simulink model "cont2_nrz_v8"  (R2016b)
settings: Solver=ode23t  StartTime=0.0  StopTime=L  FixedStep=1  RelTol=1e-6  AbsTol=1e-6
values from neighbouring files (symbols this model uses):
  a = amp(compt)    [QPSK.m]
  fin = fin_bin/Nfft    (= 0.00079345703125)    [DS_TB.m]    (also in Trace_RC.m)
settings Model: ExtModeTrigMode=oneshot  ExtModeArmWhenConnect=off  ExtModeAutoUpdateStatusClock=off  Creator=sigma  LastModifiedBy=charles
settings DataIOCC: SaveFormat=Array  SignalLoggingSaveFormat=ModelDataLogs  SaveOutput=off  SaveTime=off  SignalLoggingName=sigsOut
settings OptimizationCC: BooleanDataType=off  ExpressionDepthLimit=2147483647  InitFltsAndDblsToZero=on  LifeSpan=inf
settings DebuggingCC: SaveWithParameterizedLinksMsg=none  UnderspecifiedInitializationDetection=Classic  MergeDetectMultiDrivingBlocksExec=none  SignalResolutionControl=TryResolveAllWithWarning  MultiTaskDSMMsg=warning  MultiTaskCondExecSysMsg=none  FcnCallInpInsideContextMsg=warning  StateNameClashWarn=warning  SFUnexpectedBacktrackingDiag=warning  SFNoUnconditionalDefaultTransitionDiag=warning  SFExecutionAtInitializationDiag=none
settings HardwareCC: ProdBitPerPointer=32  ProdBitPerSizeT=32  ProdBitPerPtrDiffT=32  ProdLargestAtomicFloat=None  ProdIntDivRoundTo=Undefined  ProdEndianess=Unspecified  ProdWordSize=32  ProdHWDeviceType=32-bit Generic  TargetUnknown=on
settings ModelReferenceCC: PropagateSignalLabelsOutOfModel=off
settings RTWCC: TemplateMakefile=grt_unix.tmf
settings GRTTargetCC: TargetLangStandard=C89/C90 (ANSI)  ModelReferenceCompliant=off  ParMdlRefBuildCompliant=off  CompOptLevelCompliant=off  ConcurrentExecutionCompliant=off  CombineOutputUpdateFcns=off  MatFileLogging=off  MATLABClassNameForMDSCustomization=Simulink.SoftwareTarget.TargetSpecificTriggerConfigurationBase  GRTInterface=on
settings ConfigComp: CovMetricSettings=dw  CovHtmlReporting=on  CovSaveCumulativeToWorkspaceVar=on  CovSaveSingleToWorkspaceVar=on  CovExternalEMLEnable=off

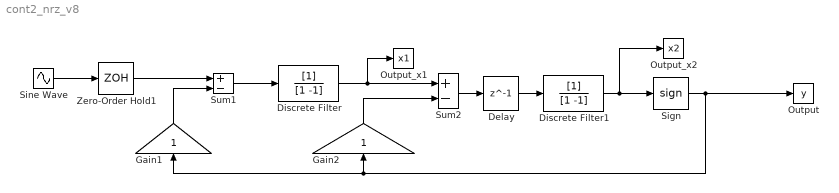
== system cont2_nrz_v8 ==
  Delay : Delay  DelayLength=1  SampleTime=1
  Discrete Filter : DiscreteFilter  Denominator=[1 -1]  SampleTime=1
  Discrete Filter1 : DiscreteFilter  Denominator=[1 -1]  SampleTime=1
  Gain1 : Gain  SaturateOnIntegerOverflow=on  OutDataTypeStr=Inherit: Same as input  ParamDataTypeStr=Inherit: Same as input
  Gain2 : Gain  SaturateOnIntegerOverflow=on  OutDataTypeStr=Inherit: Same as input  ParamDataTypeStr=Inherit: Same as input
  Output : ToWorkspace  VariableName=y  SampleTime=1
      settings: MaxDataPoints=N
  Output_x1 : ToWorkspace  VariableName=x1  SampleTime=1
      settings: MaxDataPoints=N
  Output_x2 : ToWorkspace  VariableName=x2  SampleTime=1
      settings: MaxDataPoints=N
  Sign : Signum
  Sine Wave : Sin  Amplitude=a  Frequency=2*pi*fin  SampleTime=0
  Sum1 : Sum  Inputs=+-  SaturateOnIntegerOverflow=on  InputSameDT=on  OutDataTypeStr=Inherit: Same as first input
  Sum2 : Sum  Inputs=+-  SaturateOnIntegerOverflow=on  InputSameDT=on  OutDataTypeStr=Inherit: Same as first input
  Zero-Order Hold1 : ZeroOrderHold
  wires:
  Gain1/1 -> Sum1/2
  Sine Wave/1 -> Zero-Order Hold1/1
  Gain2/1 -> Sum2/2
  Sign/1 -> Gain1/1, Gain2/1, Output/1
  Zero-Order Hold1/1 -> Sum1/1
  Discrete Filter1/1 -> Sign/1, Output_x2/1
  Discrete Filter/1 -> Sum2/1, Output_x1/1
  Sum1/1 -> Discrete Filter/1
  Sum2/1 -> Delay/1
  Delay/1 -> Discrete Filter1/1
